simulink model "kinematics_simulation"  (R2024b)
settings: Solver=FixedStepAuto  StartTime=0.0  StopTime=120  FixedStep=simulation_time_step  RelTol=1e-3
values from neighbouring files (symbols this model uses):
  T_ge_des_dataset = zeros(4, 4, num_pose_des)    [generate_poses_dataset.m]
  waypoints = [waypoints; shortenedPath.States(2:end, :)]    [path_planning.m]    (also in waypoints_restaurant.mat = [0.5 0.300302321128 0.511937054744 1.93000568213 1.540190599)
undefined symbols (not defined in the file or in its folder): alpha_roller, chassis_position_initial, d_wheel_g, links_arm_length, r_wheel, simulation_choice, T_ce_rest, T_ge_static, theta_arm_initial
settings Model: Creator=andre  LastModifiedBy=OEM
settings OptimizationCC: DefaultParameterBehavior=Inlined  EnhancedBackFolding=on  PassReuseOutputArgsAs=Individual arguments  ZeroExternalMemoryAtStartup=off  ZeroInternalMemoryAtStartup=off  MaxStackSize=64  OptimizeBlockOrder=speed  DifferentSizesBufferReuse=on  OptimizationCustomize=off  EfficientTunableParamExpr=on
settings DebuggingCC: ParameterTunabilityLossMsg=error
settings SFSimCC: MATLABDynamicMemAlloc=off
settings RTWCC: Description=Embedded Coder  SystemTargetFile=ert.tlc  HardwareBoard=Robot Operating System 2 (ROS 2)  TLCOptions="-aInlineSetEventsForThisBaseRateFcn=TLC_FALSE -aSuppressMultiTaskScheduler=TLC_FALSE  -aRateBasedStepFcn=0"  TemplateMakefile=ert_default_tmf  Toolchain=Colcon Tools  TargetLang=C++
settings CodeAppCC: ForceParamTrailComments=on  IgnoreCustomStorageClasses=off  OperatorAnnotations=on  SimulinkDataObjDesc=on  SFDataObjDesc=on  InsertBlockDesc=on
settings ERTTargetCC: CodeInterfacePackaging=C++ class  RootIOFormat=Structure reference

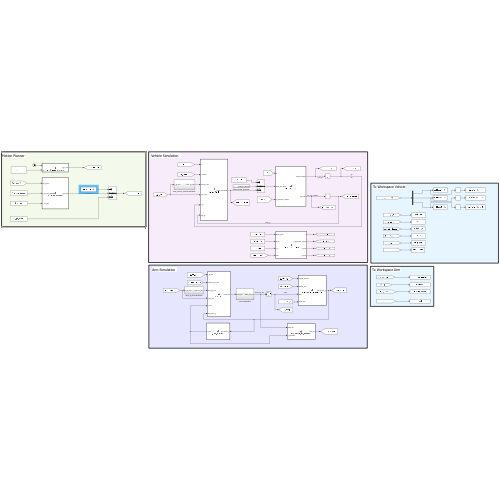
[thumbnail: Simulink's stored preview of the top-level diagram]
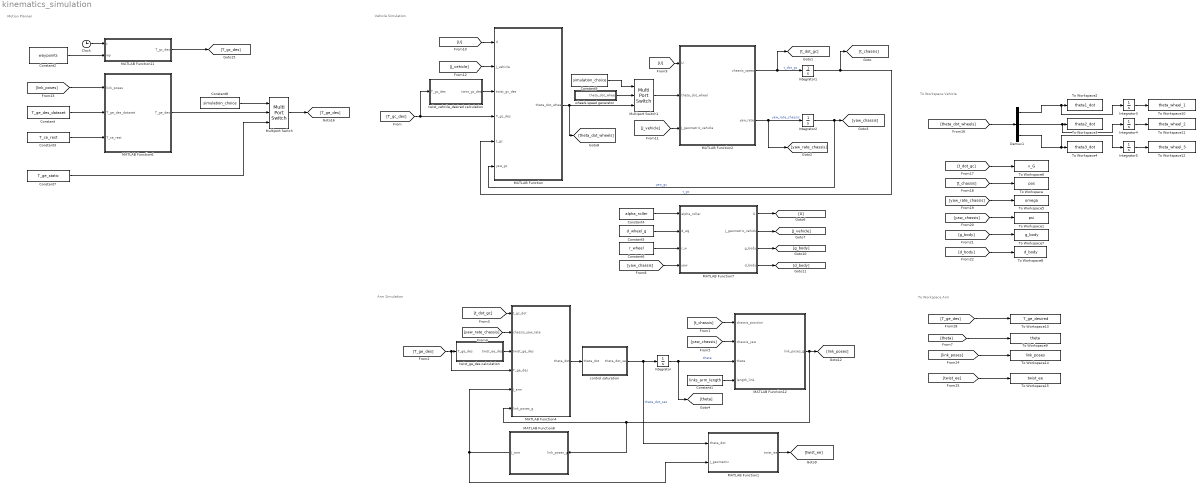
== system kinematics_simulation ==
  note: Arm Simulation
  note: To Workspace Vehicle
  note: Vehicle Simulation
  note: Motion Planner
  note: To Workspace Arm
  Clock : Clock
  Constant : Constant  Value=T_ge_des_dataset
  Constant1 : Constant  Value=links_arm_length
  Constant2 : Constant  Value=waypoints
  Constant3 : Constant  Value=T_ce_rest
  Constant4 : Constant  Value=alpha_roller
  Constant5 : Constant  Value=d_wheel_g
  Constant6 : Constant  Value=r_wheel
  Constant7 : Constant  Value=T_ge_static
  Constant8 : Constant  Value=simulation_choice
  Constant9 : Constant  Value=simulation_choice
  Demux1 : Demux  Outputs=3
  Integrator : Integrator  InitialCondition=theta_arm_initial  WrapState=on  WrappedStateUpperValue=2 * pi * ones(7,1)  WrappedStateLowerValue=zeros(7,1)
  Integrator1 : Integrator  InitialCondition=chassis_position_initial
  Integrator2 : Integrator  WrappedStateUpperValue=2*pi  WrappedStateLowerValue=0
  Integrator3 : Integrator
  Integrator4 : Integrator
  Integrator5 : Integrator
  MATLAB Function : MATLAB Function  TreatAsAtomicUnit=on
  MATLAB Function1 : MATLAB Function  TreatAsAtomicUnit=on
  MATLAB Function11 : MATLAB Function  TreatAsAtomicUnit=on
  MATLAB Function12 : MATLAB Function  TreatAsAtomicUnit=on
  MATLAB Function2 : MATLAB Function  TreatAsAtomicUnit=on
  MATLAB Function4 : MATLAB Function  TreatAsAtomicUnit=on
  MATLAB Function6 : MATLAB Function  TreatAsAtomicUnit=on
  MATLAB Function7 : MATLAB Function  TreatAsAtomicUnit=on
  MATLAB Function8 : MATLAB Function  TreatAsAtomicUnit=on
  Multiport Switch : MultiPortSwitch  Inputs=2  SaturateOnIntegerOverflow=off  InputSameDT=off
  Multiport Switch1 : MultiPortSwitch  Inputs=2  SaturateOnIntegerOverflow=off  InputSameDT=off
  To Workspace : ToWorkspace  VariableName=pos  SaveFormat=Timeseries  SampleTime=-1
  To Workspace1 : ToWorkspace  VariableName=psi  SaveFormat=Timeseries  SampleTime=-1
  To Workspace10 : ToWorkspace  VariableName=theta_wheel_1  SaveFormat=Timeseries  SampleTime=-1
  To Workspace11 : ToWorkspace  VariableName=theta_wheel_2  SaveFormat=Timeseries  SampleTime=-1
  To Workspace12 : ToWorkspace  VariableName=theta_wheel_3  SaveFormat=Timeseries  SampleTime=-1
  To Workspace13 : ToWorkspace  VariableName=T_ge_desired  SaveFormat=Timeseries  SampleTime=-1
  To Workspace14 : ToWorkspace  VariableName=link_poses  SaveFormat=Timeseries  SampleTime=-1
  To Workspace15 : ToWorkspace  VariableName=twist_ee  SaveFormat=Timeseries  SampleTime=-1
  To Workspace2 : ToWorkspace  VariableName=theta1_dot  SaveFormat=Timeseries  SampleTime=-1
  To Workspace3 : ToWorkspace  VariableName=theta2_dot  SaveFormat=Timeseries  SampleTime=-1
  To Workspace4 : ToWorkspace  VariableName=theta3_dot  SaveFormat=Timeseries  SampleTime=-1
  To Workspace5 : ToWorkspace  VariableName=omega  SaveFormat=Timeseries  SampleTime=-1
  To Workspace6 : ToWorkspace  VariableName=v_G  SaveFormat=Timeseries  SampleTime=-1
  To Workspace7 : ToWorkspace  VariableName=g_body  SaveFormat=Timeseries  SampleTime=-1
  To Workspace8 : ToWorkspace  VariableName=d_body  SaveFormat=Timeseries  SampleTime=-1
  To Workspace9 : ToWorkspace  VariableName=theta  SaveFormat=Timeseries  SampleTime=-1
  control saturation : Subsystem
  twist_ge_des calculation : Subsystem
  twist_vehcile_desired calculation : Subsystem
  wheels speed generator : Subsystem
  wires:
  MATLAB Function11/1(T_gc_des) -> [T_gc_des]
  [J_vehicle] -> MATLAB Function2/3(J_geometric_vehicle)
  [link_poses] -> To Workspace14/1
  [yaw_rate_chassis] -> To Workspace5/1
  twist_ge_des calculation/1(twist_ee_des) -> MATLAB Function4/3(twist_ge_des)
  MATLAB Function7/4(d_body) -> [d_body]
  Constant7/1 -> Multiport Switch/3
  Multiport Switch1/1 -> MATLAB Function2/2(theta_dot_wheel)
  Integrator5/1 -> To Workspace12/1
  [U] -> MATLAB Function2/1(U)
  MATLAB Function2/1(chassis_speed) -> Integrator1/1, [t_dot_gc]  "t_dot_gc"
  [yaw_chassis] -> MATLAB Function7/4(yaw)
  Integrator3/1 -> To Workspace10/1
  twist_vehcile_desired calculation/1(twist_gc_des) -> MATLAB Function/3(twist_gc_des)
  Constant6/1 -> MATLAB Function7/3(r_w)
  Integrator1/1 -> MATLAB Function/5(t_gc), [t_chassis]  "t_gc"
  Demux1/3 -> Integrator5/1, To Workspace4/1
  [T_ge_des] -> MATLAB Function4/4(T_ge_des), twist_ge_des calculation/1(T_ge_des)
  Constant2/1 -> MATLAB Function11/2(wp)
  [theta] -> To Workspace9/1
  Constant5/1 -> MATLAB Function7/2(d_wg)
  [yaw_chassis] -> MATLAB Function12/2(chassis_yaw)
  MATLAB Function2/2(yaw_rate) -> [yaw_rate_chassis], Integrator2/1  "yaw_rate_chassis"
  wheels speed generator/1(theta_dot_wheel) -> Multiport Switch1/2
  [t_dot_gc] -> MATLAB Function4/1(t_gc_dot)
  MATLAB Function7/1(U) -> [U]
  [t_chassis] -> To Workspace/1
  [d_body] -> To Workspace8/1
  [link_poses] -> MATLAB Function6/1(link_poses)
  Constant3/1 -> MATLAB Function6/3(T_ce_rest)
  Demux1/1 -> Integrator3/1, To Workspace2/1
  Clock/1 -> MATLAB Function11/1(t)
  MATLAB Function/1(theta_dot_wheel) -> [theta_dot_wheels], Multiport Switch1/3
  Integrator4/1 -> To Workspace11/1
  [t_chassis] -> MATLAB Function12/1(chassis_position)
  [J_vehicle] -> MATLAB Function/2(J_vehicle)
  Demux1/2 -> Integrator4/1, To Workspace3/1
  MATLAB Function6/1(T_ge_des) -> Multiport Switch/2
  Integrator/1 -> [theta], MATLAB Function12/3(theta)  "theta"
  Constant/1 -> MATLAB Function6/2(T_ge_des_dataset)
  MATLAB Function4/1(theta_dot) -> control saturation/1(theta_dot)
  [t_dot_gc] -> To Workspace6/1
  Constant4/1 -> MATLAB Function7/1(alpha_roller)
  [g_body] -> To Workspace7/1
  Multiport Switch/1 -> [T_ge_des]
  MATLAB Function7/2(J_geometric_vehicle) -> [J_vehicle]
  MATLAB Function1/1(twist_ee) -> [twist_ee]
  MATLAB Function12/1(link_poses_g) -> [link_poses], MATLAB Function4/6(link_poses_g), MATLAB Function8/1(link_poses_g)
  Integrator2/1 -> [yaw_chassis], MATLAB Function/6(yaw_gc)  "yaw_gc"
  [twist_ee] -> To Workspace15/1
  [T_ge_des] -> To Workspace13/1
  [yaw_rate_chassis] -> MATLAB Function4/2(chassis_yaw_rate)
  MATLAB Function7/3(g_body) -> [g_body]
  [theta_dot_wheels] -> Demux1/1
  [yaw_chassis] -> To Workspace1/1
  [T_gc_des] -> twist_vehcile_desired calculation/1(T_gc_des), MATLAB Function/4(T_gc_des)
  MATLAB Function8/1(J_arm) -> MATLAB Function1/2(J_geometric), MATLAB Function4/5(J_arm)
  Constant1/1 -> MATLAB Function12/4(length_link)
  [U] -> MATLAB Function/1(U)
  control saturation/1(theta_dot_sat) -> Integrator/1, MATLAB Function1/1(theta_dot)  "theta_dot_sat"
  Constant8/1 -> Multiport Switch/1
  Constant9/1 -> Multiport Switch1/1

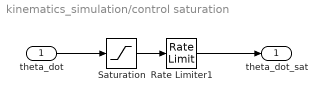
== system kinematics_simulation/control saturation ==
  theta_dot : Inport
  Rate Limiter1 : RateLimiter  RisingSlewLimit=pi/2  FallingSlewLimit=-pi/2  SampleTimeMode=inherited
  Saturation : Saturate  UpperLimit=[pi/6; pi/6; pi/6; pi/6; pi/6; pi/6; pi/12]  LowerLimit=-[pi/6; pi/6; pi/6; pi/6; pi/6; pi/6; pi/12]
  theta_dot_sat : Outport
  wires:
  Saturation/1 -> Rate Limiter1/1
  theta_dot/1 -> Saturation/1
  Rate Limiter1/1 -> theta_dot_sat/1

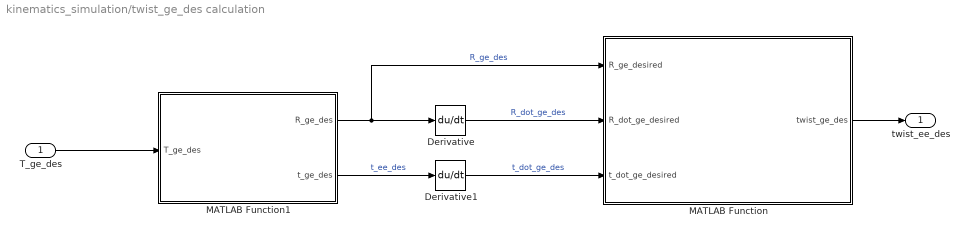
== system kinematics_simulation/twist_ge_des calculation ==
  T_ge_des : Inport
  Derivative : Derivative
  Derivative1 : Derivative
  MATLAB Function : MATLAB Function  TreatAsAtomicUnit=on
  MATLAB Function1 : MATLAB Function  TreatAsAtomicUnit=on
  twist_ee_des : Outport
  wires:
  T_ge_des/1 -> MATLAB Function1/1(T_ge_des)
  MATLAB Function1/1(R_ge_des) -> MATLAB Function/1(R_ge_desired), Derivative/1  "R_ge_des"
  Derivative/1 -> MATLAB Function/2(R_dot_ge_desired)  "R_dot_ge_des"
  MATLAB Function1/2(t_ge_des) -> Derivative1/1  "t_ee_des"
  Derivative1/1 -> MATLAB Function/3(t_dot_ge_desired)  "t_dot_ge_des"
  MATLAB Function/1(twist_ge_des) -> twist_ee_des/1

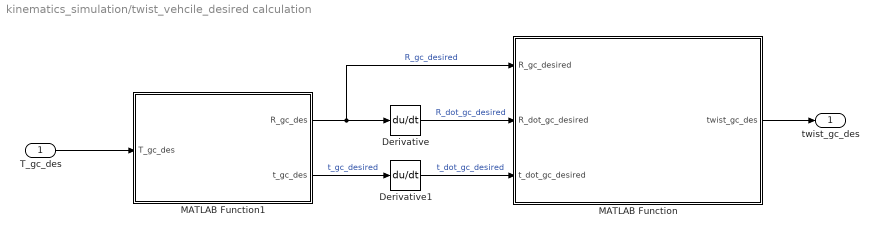
== system kinematics_simulation/twist_vehcile_desired calculation ==
  T_gc_des : Inport
  Derivative : Derivative
  Derivative1 : Derivative
  MATLAB Function : MATLAB Function  TreatAsAtomicUnit=on
  MATLAB Function1 : MATLAB Function  TreatAsAtomicUnit=on
  twist_gc_des : Outport
  wires:
  T_gc_des/1 -> MATLAB Function1/1(T_gc_des)
  MATLAB Function1/1(R_gc_des) -> MATLAB Function/1(R_gc_desired), Derivative/1  "R_gc_desired"
  Derivative/1 -> MATLAB Function/2(R_dot_gc_desired)  "R_dot_gc_desired"
  MATLAB Function1/2(t_gc_des) -> Derivative1/1  "t_gc_desired"
  Derivative1/1 -> MATLAB Function/3(t_dot_gc_desired)  "t_dot_gc_desired"
  MATLAB Function/1(twist_gc_des) -> twist_gc_des/1

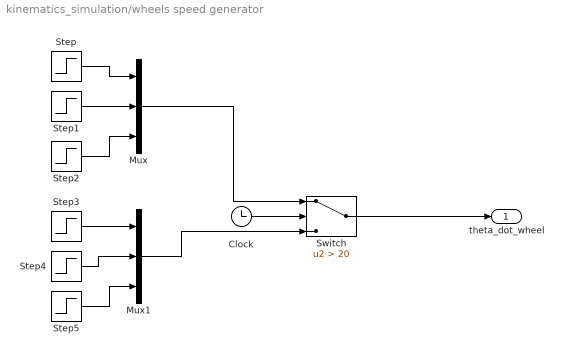
== system kinematics_simulation/wheels speed generator ==
  Clock : Clock
  Mux : Mux  Inputs=3
  Mux1 : Mux  Inputs=3
  Step : Step  Time=0  After=-5  SampleTime=0
  Step1 : Step  Time=0  After=5  SampleTime=0
  Step2 : Step  Time=0  After=5  SampleTime=0
  Step3 : Step  Time=0  After=0  SampleTime=0
  Step4 : Step  Time=0  After=0  SampleTime=0
  Step5 : Step  Time=0  After=0  SampleTime=0
  Switch : Switch  Criteria=u2 > Threshold  Threshold=20  SaturateOnIntegerOverflow=off  InputSameDT=off
  theta_dot_wheel : Outport
  wires:
  Step1/1 -> Mux/2
  Mux/1 -> Switch/1
  Step2/1 -> Mux/3
  Step/1 -> Mux/1
  Step3/1 -> Mux1/1
  Step5/1 -> Mux1/3
  Step4/1 -> Mux1/2
  Switch/1 -> theta_dot_wheel/1
  Mux1/1 -> Switch/3
  Clock/1 -> Switch/2

== matlab function kinematics_simulation/MATLAB Function8 ==
  data: link_poses_g input; J_arm output
function J_arm  = J_arm_calculation(link_poses_g)

    % Computes the geometric Jacobian from a series of transformation matrices.
    % number_of_poses - 1 (global) - 1 (chassis)  = num joints
    num_arm_links = size(link_poses_g, 3) - 1 - 1; 
    
    % ===============================
    % memory preallocation 
    % ===============================
    % Preallocate Jacobian submatrices:
    % Jv: linear velocity components (3xn)
    % Jw: angular velocity components (3xn)
    Jv = zeros(3, num_arm_links);
    Jw = zeros(3, num_arm_links);

    % Preallocate arrays for joint positions and z-axes:
    % P: positions of the joints (including the base at index 1)
    % Z: z-axis (rotation axis) of each joint
    P = zeros(3, num_arm_links+1);
    Z = zeros(3, num_arm_links+1);

    % ===============================
    % initialization
    % ===============================

    % Extract the position and z-axis for each joint from the
    % transformation matrices (link_poses_g)

    for i = 1:num_arm_links + 1 
        % The joint position is given by the fourth column of the transformation matrix
        P(:, i) = link_poses_g(1:3, 4, i+1);

        % The z-axis of the joint (rotation axis) is given by the third column of the rotation part
        Z(:, i) = link_poses_g(1:3, 3, i+1);
    end

    % Compute the end-effector position (position from the last transformation matrix)
    P_end = P(:, end);

    % =================================================
    % Geometric Jacobian calculation (chassis frame)
    % =================================================

    % Compute each column of the Jacobian:
    for i = 1:num_arm_links
        % Linear velocity component: cross product of the joint's z-axis and the vector from the joint to the end-effector
        Jv(:, i) = cross(Z(:, i), (P_end - P(:, i)));
        
        % Angular velocity component: the joint's z-axis (for revolute joints)
        Jw(:, i) = Z(:, i);
    end

    % Combine linear and angular parts into the full Jacobian (6xn)
    J_chassis = [ Jv; 
                  Jw];

    % =================================================
    % Geometric Jacobian calculation (global frame)
    % =================================================

    % A pole and reference frame is performed: chassis --> global

    T_sc = link_poses_g(:, :, 1);
    R_sc = T_sc(1:3, 1:3);
    t_sc = T_sc(1:3,   4);

    Ad_T_sc = [R_sc,    hat(t_sc)*R_sc;
               zeros(3),         R_sc];

    J_arm = Ad_T_sc * J_chassis; % global

    % =================================================
    % Check singularity
    % =================================================
    if rank(J_arm) < min(size(J_arm))
        warning('J_geometric is singular!');
    end
end

== matlab function kinematics_simulation/twist_ge_des calculation/MATLAB Function ==
  data: R_ge_desired input; R_dot_ge_desired input; twist_ge_des output; t_dot_ge_desired input
function twist_ge_des = desired_twist_ee_calculation(R_ge_desired, R_dot_ge_desired, t_dot_ge_desired)

omega_ge_des = inv_hat(R_dot_ge_desired*R_ge_desired');
twist_ge_des = [t_dot_ge_desired; omega_ge_des];

== matlab function kinematics_simulation/twist_ge_des calculation/MATLAB Function1 ==
  data: T_ge_des input; R_ge_des output; t_ge_des output
function [R_ge_des, t_ge_des]  = R_t_extraction(T_ge_des)

t_ge_des = T_ge_des(1:3, 4);
R_ge_des = T_ge_des(1:3, 1:3);

== matlab function kinematics_simulation/twist_vehcile_desired calculation/MATLAB Function ==
  data: R_gc_desired input; R_dot_gc_desired input; twist_gc_des output; t_dot_gc_desired input
function twist_gc_des = desired_twist_gc_calculation(R_gc_desired, R_dot_gc_desired, t_dot_gc_desired)

omega_d = inv_hat(R_dot_gc_desired*R_gc_desired');
twist_gc_des = [t_dot_gc_desired; omega_d];

== matlab function kinematics_simulation/twist_vehcile_desired calculation/MATLAB Function1 ==
  data: T_gc_des input; R_gc_des output; t_gc_des output
function [R_gc_des, t_gc_des]  = R_t_extraction(T_gc_des)

t_gc_des = T_gc_des(1:3, 4);
R_gc_des = T_gc_des(1:3, 1:3);

== matlab function kinematics_simulation/MATLAB Function ==
  data: U input; theta_dot_wheel output; J_vehicle input; twist_gc_des input; T_gc_des input; t_gc input; yaw_gc input
function theta_dot_wheel   = vehicle_CLIK(U, J_vehicle, twist_gc_des, T_gc_des, t_gc, yaw_gc)

% =========================
% CLIK control gain
% =========================
K = [1, 0, 0;
     0, 1, 0;
     0, 0, 1]*1e-1;

% =========================
% error calculation
% =========================
% orientation error ==================================
yaw_gc_des = atan2(T_gc_des(2,1), T_gc_des(1,1));
e_orient = atan2(sin(yaw_gc_des - yaw_gc), cos(yaw_gc_des - yaw_gc));

% position error ===========================
t_gc_des = T_gc_des(1:3, 4);
e_pos = t_gc_des(1:2) - t_gc(1:2);

% total error ===========================
e = [e_pos; 
     e_orient];

twist_gc_des_resized = [twist_gc_des(1);
                        twist_gc_des(2);
                        twist_gc_des(3)];

% =========================
% CLIK formula
% =========================
theta_dot_wheel = (1/J_vehicle)*U*(twist_gc_des_resized + K*e);

== matlab function kinematics_simulation/MATLAB Function1 ==
  data: theta_dot input; twist_ee output; J_geometric input
function twist_ee  = arm_forward_diff_kinematics(theta_dot,J_geometric)

twist_ee = J_geometric * theta_dot;

== matlab function kinematics_simulation/MATLAB Function11 ==
  data: t input; T_gc_des output; wp input
function T_gc_des = vehicle_pose_generator(t, wp)
% waypoint_interpolation_manager - Interpolates trajectory between spatial waypoints and orientations.

% Total number of waypoints
num_wp = size(wp,1);

% Time duration between each waypoint (constant)
t_wp = 10;

% Compute the indices of the waypoints to interpolate between
% idx_curr: current waypoint, idx_next: next waypoint
idx_curr = min(floor(t / t_wp) + 1, num_wp);       % ensures idx_curr does not exceed the last waypoint
idx_next = min(idx_curr + 1, num_wp);              % idx_next is the next waypoint, but not beyond the last one

% Compute the interpolation parameter (alpha in [0,1])
% Represents how close we are to the next waypoint
alpha = min(mod(t, t_wp) / t_wp, 1);

% Linear interpolation of positions
p_curr = wp(idx_curr,1:3)';  % position of the current waypoint
p_next = wp(idx_next,1:3)';  % position of the next waypoint
pos = (1 - alpha) * p_curr + alpha * p_next;  % linear interpolation (LERP)

% Interpolation of quaternions 
q_curr = wp(idx_curr,4:7)';  % quaternion of the current waypoint
q_next = wp(idx_next,4:7)';  % quaternion of the next waypoint
q_interp = (1 - alpha) * q_curr + alpha * q_next;  % linear interpolation between quaternions (LERP)
q_interp = q_interp / norm(q_interp);              % normalization to obtain a unit quaternion

% Extract interpolated quaternion components
qw = q_interp(1);  
qx = q_interp(2);  
qy = q_interp(3);  
qz = q_interp(4);  

% Convert quaternion to 3x3 rotation matrix (from qw, qx, qy, qz)
R = [1 - 2*(qy^2 + qz^2),     2*(qx*qy - qz*qw),     2*(qx*qz + qy*qw);
     2*(qx*qy + qz*qw),       1 - 2*(qx^2 + qz^2),   2*(qy*qz - qx*qw);
     2*(qx*qz - qy*qw),       2*(qy*qz + qx*qw),     1 - 2*(qx^2 + qy^2)];

T_gc_des = [R, pos;
            0 0 0 1];
end

== matlab function kinematics_simulation/MATLAB Function12 ==
  data: chassis_position input; chassis_yaw input; theta input; link_poses_g output; length_link input
function link_poses_g  = arm_forward_kinematics_DH(chassis_position, chassis_yaw, theta, length_link)

    DH_table = [
       length_link(1),  theta(1),  0,  -pi/2;
       length_link(2),  theta(2),  0,   pi/2;
       length_link(3),  theta(3),  0,   pi/2;
       length_link(4),  theta(4),  0,  -pi/2;
       length_link(5),  theta(5),  0,  -pi/2;
       length_link(6),  theta(6),  0,   pi/2;
       length_link(7),  theta(7),  0,   0;
    ];
    
    % Computes forward kinematics given the DH table and joint angles.
    n = size(DH_table, 1);         % Number of joints

    % Preallocate transformation matrices (n joints + 1 chassis + 1 global)
    link_poses_g = zeros(4, 4, n+1+1); 
    
    % ===================================
    % Add world RFs
    % ===================================

    link_poses_g(:, :, 1) = eye(4);

    % ===================================
    % Add chassis RFs
    % ===================================
    
    % Initial transformation matrix (chassis pose relative to global)
    R_gc = [cos(chassis_yaw), -sin(chassis_yaw), 0;
            sin(chassis_yaw),  cos(chassis_yaw), 0;
                           0,                 0, 1];

    t_gc = [chassis_position(1);
            chassis_position(2);
            chassis_position(3)];

    T_gc = [R_gc, t_gc;
            0, 0, 0, 1];

    link_poses_g(:, :, 2) = T_gc;

    % ===================================
    % Add arm joints RFs
    % ===================================

    T_past = T_gc;
    
    % Compute forward kinematics
    for i = 1:n
        d = DH_table(i, 1); 
        theta = DH_table(i, 2);               
        a = DH_table(i, 3);                       
        alpha = DH_table(i, 4);             
    
        % Transformation matrix following DH convention
        Ai = [
            cos(theta), -sin(theta)*cos(alpha),  sin(theta)*sin(alpha), a*cos(theta);
            sin(theta),  cos(theta)*cos(alpha), -cos(theta)*sin(alpha), a*sin(theta);
            0,           sin(alpha),             cos(alpha),            d;
            0,           0,                      0,                     1
        ];
    
        % Update the total transformation
        T_past = T_past * Ai;
    
        % Store the partial transformation
        link_poses_g(:, :, i+1+1) = T_past; % +1+1 skip global and chassis
    end
end

== matlab function kinematics_simulation/MATLAB Function2 ==
  data: U input; theta_dot_wheel input; J_geometric_vehicle input; chassis_speed output; yaw_rate output
function [chassis_speed, yaw_rate] = vehicle_kinematics(U, theta_dot_wheel, J_geometric_vehicle)

% ===========================================
% robot twist (spatial coordinates)
% ===========================================
twist_spatial = pinv(U)*(J_geometric_vehicle * theta_dot_wheel); 

twist_S = [twist_spatial(1);
           twist_spatial(2);
           0;
           0;
           0;
           twist_spatial(3)];

chassis_speed = twist_S(1:3);  
yaw_rate = twist_S(6);         % chassis yaw rate

== matlab function kinematics_simulation/MATLAB Function4 ==
  data: t_gc_dot input; chassis_yaw_rate input; twist_ge_des input; T_ge_des input; theta_dot output; J_arm input; link_poses_g input
function theta_dot   = Arm_CLIK(t_gc_dot, chassis_yaw_rate, twist_ge_des, T_ge_des, J_arm, link_poses_g)

% =========================
% desired ee twist calculation
% =========================
t_ge_dot_desired = twist_ge_des(1:3);
omega_ge_des = twist_ge_des(4:6);


% =========================
% error calculation
% =========================
% orientation error ===========================
% desired end effector pose relative to global
R_ge_des = T_ge_des(1:3, 1:3);
Q_ge_des = rotm2quat(R_ge_des);  % Convert rotation matrix to quaternion
eta_ge_des = Q_ge_des(1);        % Scalar part
epsilon_ge_des = Q_ge_des(2:4)'; % Vector part

% end effector pose relative to global
T_ge = link_poses_g(:, :, end);
R_ge = T_ge(1:3, 1:3);
Q_ge = rotm2quat(R_ge);   % Convert rotation matrix to quaternion
eta_ge = Q_ge(1);         % Scalar part
epsilon_ge = Q_ge(2:4)';  % Vector part

e_orientation = eta_ge*epsilon_ge_des - eta_ge_des*epsilon_ge - hat(epsilon_ge_des)*epsilon_ge;

% position error ===========================
t_ge_des = T_ge_des(1:3, 4);
t_ge = T_ge(1:3, 4);
e_position = t_ge_des - t_ge;


% =========================
% CLIK control gain
% =========================
K_p = eye(3)*3e-1;
K_o_base = 8e-1; % base orientation gain

% Adaptive K_o
e_orientation_norm = norm(e_orientation);

% scaling law (smooth transition)
k_scale = min(15, K_o_base + 200*e_orientation_norm);  
K_o = eye(3)* k_scale * K_o_base;  % adaptive K_o


% ===========================================
% chassis movement feedforward compensation
% ===========================================
% rotation compensation
omega_ge_transport = [0; 0; chassis_yaw_rate];

% speed compensation
T_gc = link_poses_g(:, :, 2);
t_gc = T_gc(1:3, 4);
t_ce = t_ge - t_gc;
t_ge_dot_transport =  t_gc_dot + cross(omega_ge_transport, t_ce);


% =========================
% Task priority CLIK
% =========================
% Compute desired errors
t_ge_dot_error = t_ge_dot_desired - t_ge_dot_transport + K_p * e_position;
omega_ge_error = omega_ge_des - omega_ge_transport +  K_o * e_orientation;

% Define Jacobians for orientation and position
J_o = J_arm(4:6,:);
J_p = J_arm(1:3,:);

% High priority task (orientation)
theta_dot_orientation = pinv(J_o) * omega_ge_error;

% Low priority task (position)
% Compute nullspace projector
N = eye(size(J_arm,2)) - pinv(J_o) * J_o;

theta_dot_position = pinv(J_p * N) * t_ge_dot_error;

% =========================
% Error saturation
% =========================
saturation_speed_rot = 0.7;
saturation_speed_trasl = 0.7;
for joint_index = 1:length(theta_dot_position)
    % ----------
    if theta_dot_orientation(joint_index) > saturation_speed_rot
        theta_dot_orientation(joint_index) = saturation_speed_rot;
    end
    if theta_dot_orientation(joint_index) < -saturation_speed_rot
        theta_dot_orientation(joint_index) = -saturation_speed_rot;
    end
    % ----------
    if theta_dot_position(joint_index) > saturation_speed_trasl
        theta_dot_position(joint_index) = saturation_speed_trasl;
    end
    if theta_dot_position(joint_index) < -saturation_speed_trasl
        theta_dot_position(joint_index) = -saturation_speed_trasl;
    end
    
end

% =========================
% Speed calculation
% =========================
theta_dot = theta_dot_orientation + N * theta_dot_position;

== matlab function kinematics_simulation/MATLAB Function6 ==
  data: link_poses input; T_ge_des output; T_ge_des_dataset input; T_ce_rest input
function T_ge_des   = arm_pose_generator(link_poses, T_ge_des_dataset, T_ce_rest)

T_gc = link_poses(:, :, 2);
t_gc = T_gc(1:3, 4);

arm_reach = 1;

% rest pose
T_ge_des = T_gc * T_ce_rest;


% client reach pose
for pose_index = 1:size(T_ge_des_dataset,3)

    T_ge_des_candidate = T_ge_des_dataset(:, :, pose_index);
    t_ge_des_candidate = T_ge_des_candidate(1:3, 4);
    
    if norm(t_gc - t_ge_des_candidate) > arm_reach
        continue % out of reach position
    end
    
    % inside reach position
    T_ge_des = T_ge_des_candidate;
    break

end

== matlab function kinematics_simulation/MATLAB Function7 ==
  data: alpha_roller input; d_wg input; r_w input; yaw input; U output; J_geometric_vehicle output; g_body output; d_body output
function [U, J_geometric_vehicle, g_body, d_body] = vehicle_params_calculation(alpha_roller, d_wg, r_w, yaw)

% d_wg: distance: wheel axis --> COM vehicle
% r_w: wheel radius
% alpha_roller: rollers angle

% ===========================================
% distance G --> carrier center (body frame)
% ===========================================
d1_body = d_wg*[1; 
                0];

d2_body = d_wg*[-sin(deg2rad(30)); 
                 cos(deg2rad(30))]; 

d3_body = d_wg*[-sin(deg2rad(30)); 
                -cos(deg2rad(30))]; 

% ===========================================
% roller axis (body frame)
% ===========================================
g1_body = [-cos(alpha_roller); 
           -sin(alpha_roller)];

g2_body = [ cos(deg2rad(60) - alpha_roller); 
           -sin(deg2rad(60) - alpha_roller)];

g3_body = [cos(deg2rad(60) + alpha_roller); 
           sin(deg2rad(60) + alpha_roller)];

g_body = [g1_body; g2_body; g3_body];
d_body = [d1_body; d2_body; d3_body];


% ==========================================
% Body --> Spatial
% ==========================================
R_sb = [cos(yaw), -sin(yaw);
        sin(yaw),  cos(yaw)];

g1_spatial = R_sb * g1_body;
g2_spatial = R_sb * g2_body;
g3_spatial = R_sb * g3_body;

d1_spatial = R_sb * d1_body;
d2_spatial = R_sb * d2_body;
d3_spatial = R_sb * d3_body;
 
% ==========================================
% J * theta_dot = U * Xi
% ==========================================
E = [0, -1;
     1,  0];

U = [g1_spatial', g1_spatial' * E * d1_spatial;
     g2_spatial', g2_spatial' * E * d2_spatial;
     g3_spatial', g3_spatial' * E * d3_spatial];

% ==========================================
% Geometric Jacobian 
% ==========================================
J_geometric_vehicle = -r_w*sin(alpha_roller);
